simulink model "Correct_ESC_Model_with_Motor_Quadcopter_E2A"  (R2018b)
settings: Solver=VariableStepAuto  StartTime=0.0  StopTime=10  RelTol=1e-3
settings Model: Creator=hermansoyfer  LastModifiedBy=tdarrah
settings SFSimCC: SimUseLocalCustomCode=off
settings RTWCC: RTWUseLocalCustomCode=off
settings CodeAppCC: StateflowObjectComments=on

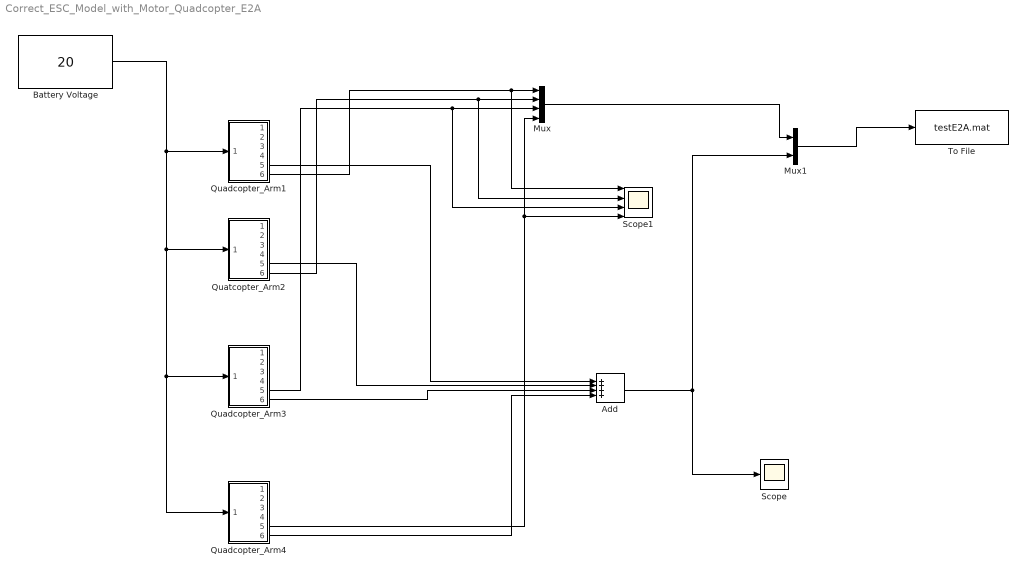
== system Correct_ESC_Model_with_Motor_Quadcopter_E2A ==
  Add : Sum  Inputs=++++
  Battery Voltage : Constant  Value=20
  Mux : Mux
  Mux1 : Mux  Inputs=2
  Quadcopter_Arm1 : Subsystem
  Quadcopter_Arm3 : Subsystem
  Quadcopter_Arm4 : Subsystem
  Quatcopter_Arm2 : Subsystem
  Scope : Scope
  Scope1 : Scope  NumInputPorts=4
  To File : ToFile  Filename=testE2A.mat  MatrixName=Data
  wires:
  Battery Voltage/1 -> Quadcopter_Arm1/1(In1), Quatcopter_Arm2/1(In1), Quadcopter_Arm3/1(In1), Quadcopter_Arm4/1(In1)
  Quadcopter_Arm1/5(M1Current) -> Add/1
  Quatcopter_Arm2/5(M2Current) -> Add/2
  Quadcopter_Arm3/6(M3Current) -> Add/3
  Quadcopter_Arm4/6(M4Current) -> Add/4
  Add/1 -> Mux1/2, Scope/1
  Quadcopter_Arm1/6(M1Voltage) -> Scope1/1, Mux/1
  Quatcopter_Arm2/6(M2Voltatge) -> Scope1/2, Mux/2
  Quadcopter_Arm3/5(M3Voltage) -> Scope1/3, Mux/3
  Quadcopter_Arm4/5(M4Voltage) -> Scope1/4, Mux/4
  Mux/1 -> Mux1/1
  Mux1/1 -> To File/1

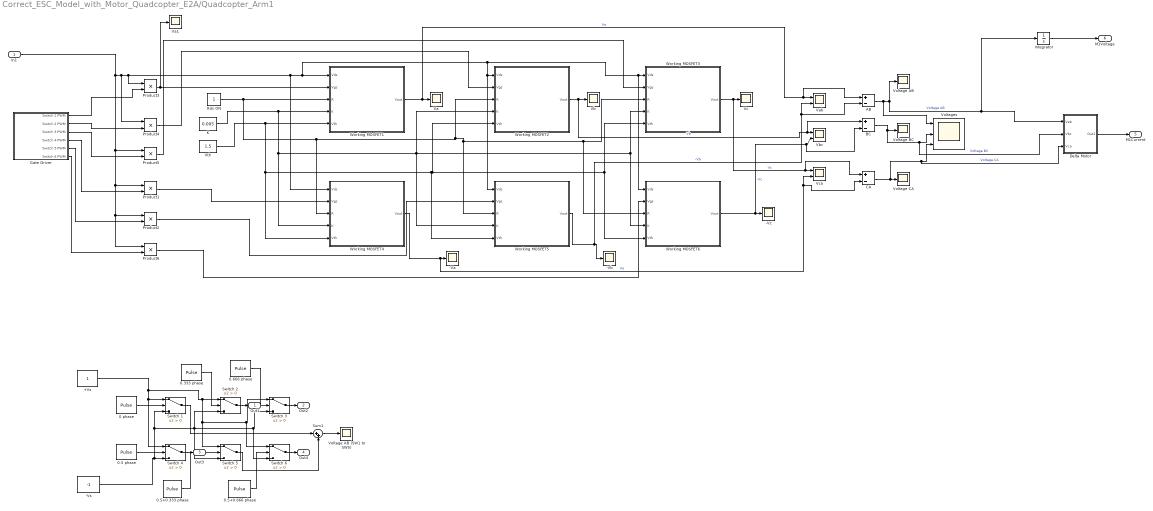
== system Correct_ESC_Model_with_Motor_Quadcopter_E2A/Quadcopter_Arm1 ==
  In1 : Inport
  +Vs : Constant
  -Va : Scope
  -Vb : Scope
  -Vc : Scope
  -Vs : Constant  Value=-1
  0 phase : DiscretePulseGenerator  PulseType=Time based  Period=1  PulseWidth=50
  0.333 phase : DiscretePulseGenerator  PulseType=Time based  Period=1  PulseWidth=50  PhaseDelay=1/3
  0.5 phase : DiscretePulseGenerator  PulseType=Time based  Period=1  PulseWidth=50  PhaseDelay=.5
  0.5+0.333 phase : DiscretePulseGenerator  PulseType=Time based  Period=1  PulseWidth=50  PhaseDelay=0.5 + 1/3
  0.5+0.666 phase : DiscretePulseGenerator  PulseType=Time based  Period=1  PulseWidth=50  PhaseDelay=2/3+0.5
  0.666 phase : DiscretePulseGenerator  PulseType=Time based  Period=1  PulseWidth=50  PhaseDelay=2/3
  AB : Sum  Inputs=+-
  BC : Sum  Inputs=+-
  CA : Sum  Inputs=+-
  Delta Motor : Subsystem
  Gate Driver : Subsystem
  Integrator : Integrator
  K : Constant  Value=0.005
  Product{1..6} (6 alike) : Product
  Rds ON : Constant
  Sum1 : Sum  Inputs=|++
  Switch {1..6} (6 alike) : Switch  Criteria=u2 > Threshold
  Va : Scope
  Va1 : Scope
  Vab : Scope  NumInputPorts=2
  Vb : Scope
  Vbc : Scope  NumInputPorts=2
  Vc : Scope
  Vca : Scope  NumInputPorts=2
  Voltage AB : Scope
  Voltage AB (SW1 to SW5) : Scope
  Voltage BC : Scope
  Voltage CA : Scope
  Voltages : Scope  NumInputPorts=3
  Vth : Constant  Value=1.5
  Working MOSFET1 : MATLAB Function  TreatAsAtomicUnit=on
  Working MOSFET2 : MATLAB Function  TreatAsAtomicUnit=on
  Working MOSFET3 : MATLAB Function  TreatAsAtomicUnit=on
  Working MOSFET4 : MATLAB Function  TreatAsAtomicUnit=on
  Working MOSFET5 : MATLAB Function  TreatAsAtomicUnit=on
  Working MOSFET6 : MATLAB Function  TreatAsAtomicUnit=on
  Out1 : Outport
  Out2 : Outport  Port=2
  Out3 : Outport  Port=3
  Out4 : Outport  Port=4
  M1Current : Outport  Port=5
  M1Voltage : Outport  Port=6
  wires:
  Switch 5/1 -> Sum1/2
  Working MOSFET4/1(Vout) -> CA/2, Vca/2, -Va/1  "Va"
  Working MOSFET6/1(Vout) -> BC/2, Vbc/2, -Vc/1  "-Vc"
  AB/1 -> Voltages/1, Integrator/1, Delta Motor/1(Vab), Voltage AB/1  "Voltage AB"
  In1/1 -> Product6/1, Product2/1, Product1/1, Product5/1, Product4/1, Working MOSFET4/1(Vds), Working MOSFET6/1(Vds), Working MOSFET3/1(Vds), Working MOSFET5/1(Vds), Working MOSFET2/1(Vds), Working MOSFET1/1(Vds), Product3/1
  K/1 -> Working MOSFET4/4(K), Working MOSFET5/4(K), Working MOSFET2/4(K), Working MOSFET6/4(K), Working MOSFET3/4(K), Working MOSFET1/4(K)
  Product5/1 -> Working MOSFET3/2(Vgs)
  0.5+0.333 phase/1 -> Switch 5/2
  Gate Driver/3(Switch 3 PWM) -> Product5/2
  Gate Driver/6(Switch 6 PWM) -> Product6/2
  Working MOSFET5/1(Vout) -> AB/2, Vab/2, -Vb/1  "-Vb"
  Gate Driver/5(Switch 5 PWM) -> Product2/2
  Working MOSFET1/1(Vout) -> AB/1, Vab/1, Va/1  "Va"
  0 phase/1 -> Switch 1/2
  Gate Driver/2(Switch 2 PWM) -> Product4/2
  Gate Driver/4(Switch 4 PWM) -> Product1/2
  BC/1 -> Delta Motor/2(Vbc), Voltages/2, Voltage BC/1  "Voltage BC"
  CA/1 -> Delta Motor/3(Vca), Voltages/3, Voltage CA/1  "Voltage CA"
  Working MOSFET3/1(Vout) -> CA/1, Vca/1, Vc/1  "Vc"
  Vth/1 -> Working MOSFET4/5(Vth), Working MOSFET5/5(Vth), Working MOSFET2/5(Vth), Working MOSFET6/5(Vth), Working MOSFET3/5(Vth), Working MOSFET1/5(Vth)
  Product1/1 -> Working MOSFET4/2(Vgs)
  0.333 phase/1 -> Switch 2/2
  Sum1/1 -> Voltage AB (SW1 to SW5)/1
  0.5 phase/1 -> Switch 4/2
  Switch 1/1 -> Sum1/1
  Working MOSFET2/1(Vout) -> BC/1, Vbc/1, Vb/1  "Vb"
  Switch 6/1 -> Out4/1
  Switch 2/1 -> Out1/1
  Switch 4/1 -> Out3/1
  Product2/1 -> Working MOSFET5/2(Vgs)
  Switch 3/1 -> Out2/1
  +Vs/1 -> Switch 6/1, Switch 3/1, Switch 5/1, Switch 2/1, Switch 4/1, Switch 1/1
  0.666 phase/1 -> Switch 3/2
  0.5+0.666 phase/1 -> Switch 6/2
  -Vs/1 -> Switch 1/3, Switch 6/3, Switch 3/3, Switch 2/3, Switch 5/3, Switch 4/3
  Rds ON/1 -> Working MOSFET1/3(R), Working MOSFET4/3(R), Working MOSFET3/3(R), Working MOSFET6/3(R), Working MOSFET5/3(R), Working MOSFET2/3(R)
  Product4/1 -> Working MOSFET2/2(Vgs)
  Product3/1 -> Working MOSFET1/2(Vgs), Va1/1
  Product6/1 -> Working MOSFET6/2(Vgs)
  Delta Motor/1(Out1) -> M1Current/1
  Integrator/1 -> M1Voltage/1
  Gate Driver/1(Switch 1 PWM) -> Product3/2

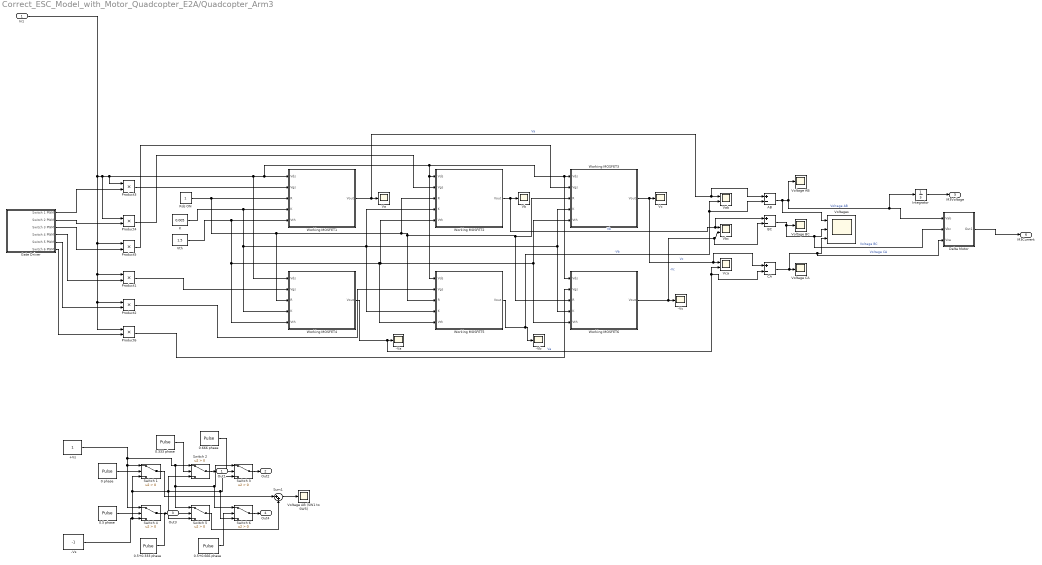
== system Correct_ESC_Model_with_Motor_Quadcopter_E2A/Quadcopter_Arm3 ==
  In1 : Inport
  +Vs : Constant
  -Va : Scope
  -Vb : Scope
  -Vc : Scope
  -Vs : Constant  Value=-1
  0 phase : DiscretePulseGenerator  PulseType=Time based  Period=1  PulseWidth=50
  0.333 phase : DiscretePulseGenerator  PulseType=Time based  Period=1  PulseWidth=50  PhaseDelay=1/3
  0.5 phase : DiscretePulseGenerator  PulseType=Time based  Period=1  PulseWidth=50  PhaseDelay=.5
  0.5+0.333 phase : DiscretePulseGenerator  PulseType=Time based  Period=1  PulseWidth=50  PhaseDelay=0.5 + 1/3
  0.5+0.666 phase : DiscretePulseGenerator  PulseType=Time based  Period=1  PulseWidth=50  PhaseDelay=2/3+0.5
  0.666 phase : DiscretePulseGenerator  PulseType=Time based  Period=1  PulseWidth=50  PhaseDelay=2/3
  AB : Sum  Inputs=+-
  BC : Sum  Inputs=+-
  CA : Sum  Inputs=+-
  Delta Motor : Subsystem
  Gate Driver : Subsystem
  Integrator : Integrator
  K : Constant  Value=0.005
  Product{1..6} (6 alike) : Product
  Rds ON : Constant
  Sum1 : Sum  Inputs=|++
  Switch {1..6} (6 alike) : Switch  Criteria=u2 > Threshold
  Va : Scope
  Vab : Scope  NumInputPorts=2
  Vb : Scope
  Vbc : Scope  NumInputPorts=2
  Vc : Scope
  Vca : Scope  NumInputPorts=2
  Voltage AB : Scope
  Voltage AB (SW1 to SW5) : Scope
  Voltage BC : Scope
  Voltage CA : Scope
  Voltages : Scope  NumInputPorts=3
  Vth : Constant  Value=1.5
  Working MOSFET1 : MATLAB Function  TreatAsAtomicUnit=on
  Working MOSFET2 : MATLAB Function  TreatAsAtomicUnit=on
  Working MOSFET3 : MATLAB Function  TreatAsAtomicUnit=on
  Working MOSFET4 : MATLAB Function  TreatAsAtomicUnit=on
  Working MOSFET5 : MATLAB Function  TreatAsAtomicUnit=on
  Working MOSFET6 : MATLAB Function  TreatAsAtomicUnit=on
  Out1 : Outport
  Out2 : Outport  Port=2
  Out3 : Outport  Port=3
  Out4 : Outport  Port=4
  M3Voltage : Outport  Port=5
  M3Current : Outport  Port=6
  wires:
  Switch 5/1 -> Sum1/2
  Working MOSFET4/1(Vout) -> CA/2, Vca/2, -Va/1  "Va"
  Working MOSFET6/1(Vout) -> BC/2, Vbc/2, -Vc/1  "-Vc"
  AB/1 -> Voltages/1, Integrator/1, Delta Motor/1(Vab), Voltage AB/1  "Voltage AB"
  In1/1 -> Product6/1, Product2/1, Product1/1, Product5/1, Product4/1, Working MOSFET4/1(Vds), Working MOSFET6/1(Vds), Working MOSFET3/1(Vds), Working MOSFET5/1(Vds), Working MOSFET2/1(Vds), Working MOSFET1/1(Vds), Product3/1
  K/1 -> Working MOSFET4/4(K), Working MOSFET5/4(K), Working MOSFET2/4(K), Working MOSFET6/4(K), Working MOSFET3/4(K), Working MOSFET1/4(K)
  Product5/1 -> Working MOSFET3/2(Vgs)
  0.5+0.333 phase/1 -> Switch 5/2
  Gate Driver/3(Switch 3 PWM) -> Product5/2
  Gate Driver/6(Switch 6 PWM) -> Product6/2
  Working MOSFET5/1(Vout) -> AB/2, Vab/2, -Vb/1  "-Vb"
  Gate Driver/5(Switch 5 PWM) -> Product2/2
  Working MOSFET1/1(Vout) -> AB/1, Vab/1, Va/1  "Va"
  0 phase/1 -> Switch 1/2
  Gate Driver/2(Switch 2 PWM) -> Product4/2
  Gate Driver/4(Switch 4 PWM) -> Product1/2
  BC/1 -> Delta Motor/2(Vbc), Voltages/2, Voltage BC/1  "Voltage BC"
  CA/1 -> Delta Motor/3(Vca), Voltages/3, Voltage CA/1  "Voltage CA"
  Working MOSFET3/1(Vout) -> CA/1, Vca/1, Vc/1  "Vc"
  Gate Driver/1(Switch 1 PWM) -> Product3/2
  Vth/1 -> Working MOSFET4/5(Vth), Working MOSFET5/5(Vth), Working MOSFET2/5(Vth), Working MOSFET6/5(Vth), Working MOSFET3/5(Vth), Working MOSFET1/5(Vth)
  Product1/1 -> Working MOSFET4/2(Vgs)
  0.333 phase/1 -> Switch 2/2
  Sum1/1 -> Voltage AB (SW1 to SW5)/1
  0.5 phase/1 -> Switch 4/2
  Switch 1/1 -> Sum1/1
  Working MOSFET2/1(Vout) -> BC/1, Vbc/1, Vb/1  "Vb"
  Switch 6/1 -> Out4/1
  Switch 2/1 -> Out1/1
  Switch 4/1 -> Out3/1
  Product2/1 -> Working MOSFET5/2(Vgs)
  Switch 3/1 -> Out2/1
  +Vs/1 -> Switch 6/1, Switch 3/1, Switch 5/1, Switch 2/1, Switch 4/1, Switch 1/1
  0.666 phase/1 -> Switch 3/2
  0.5+0.666 phase/1 -> Switch 6/2
  -Vs/1 -> Switch 1/3, Switch 6/3, Switch 3/3, Switch 2/3, Switch 5/3, Switch 4/3
  Rds ON/1 -> Working MOSFET1/3(R), Working MOSFET4/3(R), Working MOSFET3/3(R), Working MOSFET6/3(R), Working MOSFET5/3(R), Working MOSFET2/3(R)
  Product4/1 -> Working MOSFET2/2(Vgs)
  Product3/1 -> Working MOSFET1/2(Vgs)
  Product6/1 -> Working MOSFET6/2(Vgs)
  Integrator/1 -> M3Voltage/1
  Delta Motor/1(Out1) -> M3Current/1

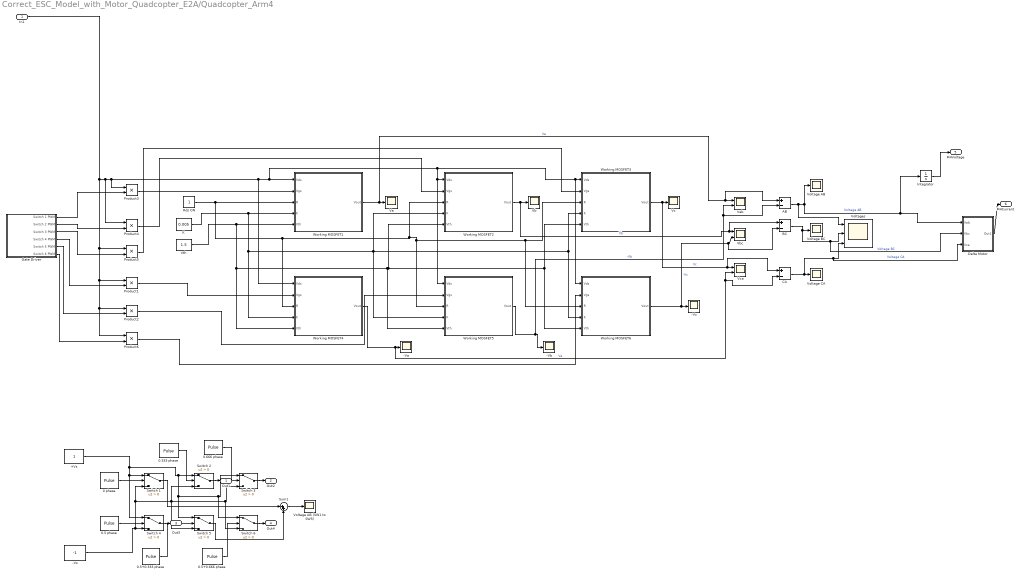
== system Correct_ESC_Model_with_Motor_Quadcopter_E2A/Quadcopter_Arm4 ==
  In1 : Inport
  +Vs : Constant
  -Va : Scope
  -Vb : Scope
  -Vc : Scope
  -Vs : Constant  Value=-1
  0 phase : DiscretePulseGenerator  PulseType=Time based  Period=1  PulseWidth=50
  0.333 phase : DiscretePulseGenerator  PulseType=Time based  Period=1  PulseWidth=50  PhaseDelay=1/3
  0.5 phase : DiscretePulseGenerator  PulseType=Time based  Period=1  PulseWidth=50  PhaseDelay=.5
  0.5+0.333 phase : DiscretePulseGenerator  PulseType=Time based  Period=1  PulseWidth=50  PhaseDelay=0.5 + 1/3
  0.5+0.666 phase : DiscretePulseGenerator  PulseType=Time based  Period=1  PulseWidth=50  PhaseDelay=2/3+0.5
  0.666 phase : DiscretePulseGenerator  PulseType=Time based  Period=1  PulseWidth=50  PhaseDelay=2/3
  AB : Sum  Inputs=+-
  BC : Sum  Inputs=+-
  CA : Sum  Inputs=+-
  Delta Motor : Subsystem
  Gate Driver : Subsystem
  Integrator : Integrator
  K : Constant  Value=0.005
  Product{1..6} (6 alike) : Product
  Rds ON : Constant
  Sum1 : Sum  Inputs=|++
  Switch {1..6} (6 alike) : Switch  Criteria=u2 > Threshold
  Va : Scope
  Vab : Scope  NumInputPorts=2
  Vb : Scope
  Vbc : Scope  NumInputPorts=2
  Vc : Scope
  Vca : Scope  NumInputPorts=2
  Voltage AB : Scope
  Voltage AB (SW1 to SW5) : Scope
  Voltage BC : Scope
  Voltage CA : Scope
  Voltages : Scope  NumInputPorts=3
  Vth : Constant  Value=1.5
  Working MOSFET1 : MATLAB Function  TreatAsAtomicUnit=on
  Working MOSFET2 : MATLAB Function  TreatAsAtomicUnit=on
  Working MOSFET3 : MATLAB Function  TreatAsAtomicUnit=on
  Working MOSFET4 : MATLAB Function  TreatAsAtomicUnit=on
  Working MOSFET5 : MATLAB Function  TreatAsAtomicUnit=on
  Working MOSFET6 : MATLAB Function  TreatAsAtomicUnit=on
  Out1 : Outport
  Out2 : Outport  Port=2
  Out3 : Outport  Port=3
  Out4 : Outport  Port=4
  M4Voltage : Outport  Port=5
  M4Current : Outport  Port=6
  wires:
  Switch 5/1 -> Sum1/2
  Working MOSFET4/1(Vout) -> CA/2, Vca/2, -Va/1  "Va"
  Working MOSFET6/1(Vout) -> BC/2, Vbc/2, -Vc/1  "-Vc"
  AB/1 -> Voltages/1, Integrator/1, Delta Motor/1(Vab), Voltage AB/1  "Voltage AB"
  In1/1 -> Product6/1, Product2/1, Product1/1, Product5/1, Product4/1, Working MOSFET4/1(Vds), Working MOSFET6/1(Vds), Working MOSFET3/1(Vds), Working MOSFET5/1(Vds), Working MOSFET2/1(Vds), Working MOSFET1/1(Vds), Product3/1
  K/1 -> Working MOSFET4/4(K), Working MOSFET5/4(K), Working MOSFET2/4(K), Working MOSFET6/4(K), Working MOSFET3/4(K), Working MOSFET1/4(K)
  Product5/1 -> Working MOSFET3/2(Vgs)
  0.5+0.333 phase/1 -> Switch 5/2
  Gate Driver/3(Switch 3 PWM) -> Product5/2
  Gate Driver/6(Switch 6 PWM) -> Product6/2
  Working MOSFET5/1(Vout) -> AB/2, Vab/2, -Vb/1  "-Vb"
  Gate Driver/5(Switch 5 PWM) -> Product2/2
  Working MOSFET1/1(Vout) -> AB/1, Vab/1, Va/1  "Va"
  0 phase/1 -> Switch 1/2
  Gate Driver/2(Switch 2 PWM) -> Product4/2
  Gate Driver/4(Switch 4 PWM) -> Product1/2
  BC/1 -> Delta Motor/2(Vbc), Voltages/2, Voltage BC/1  "Voltage BC"
  CA/1 -> Delta Motor/3(Vca), Voltages/3, Voltage CA/1  "Voltage CA"
  Working MOSFET3/1(Vout) -> CA/1, Vca/1, Vc/1  "Vc"
  Gate Driver/1(Switch 1 PWM) -> Product3/2
  Vth/1 -> Working MOSFET4/5(Vth), Working MOSFET5/5(Vth), Working MOSFET2/5(Vth), Working MOSFET6/5(Vth), Working MOSFET3/5(Vth), Working MOSFET1/5(Vth)
  Product1/1 -> Working MOSFET4/2(Vgs)
  0.333 phase/1 -> Switch 2/2
  Sum1/1 -> Voltage AB (SW1 to SW5)/1
  0.5 phase/1 -> Switch 4/2
  Switch 1/1 -> Sum1/1
  Working MOSFET2/1(Vout) -> BC/1, Vbc/1, Vb/1  "Vb"
  Switch 6/1 -> Out4/1
  Switch 2/1 -> Out1/1
  Switch 4/1 -> Out3/1
  Product2/1 -> Working MOSFET5/2(Vgs)
  Switch 3/1 -> Out2/1
  +Vs/1 -> Switch 6/1, Switch 3/1, Switch 5/1, Switch 2/1, Switch 4/1, Switch 1/1
  0.666 phase/1 -> Switch 3/2
  0.5+0.666 phase/1 -> Switch 6/2
  -Vs/1 -> Switch 1/3, Switch 6/3, Switch 3/3, Switch 2/3, Switch 5/3, Switch 4/3
  Rds ON/1 -> Working MOSFET1/3(R), Working MOSFET4/3(R), Working MOSFET3/3(R), Working MOSFET6/3(R), Working MOSFET5/3(R), Working MOSFET2/3(R)
  Product4/1 -> Working MOSFET2/2(Vgs)
  Product3/1 -> Working MOSFET1/2(Vgs)
  Product6/1 -> Working MOSFET6/2(Vgs)
  Integrator/1 -> M4Voltage/1
  Delta Motor/1(Out1) -> M4Current/1

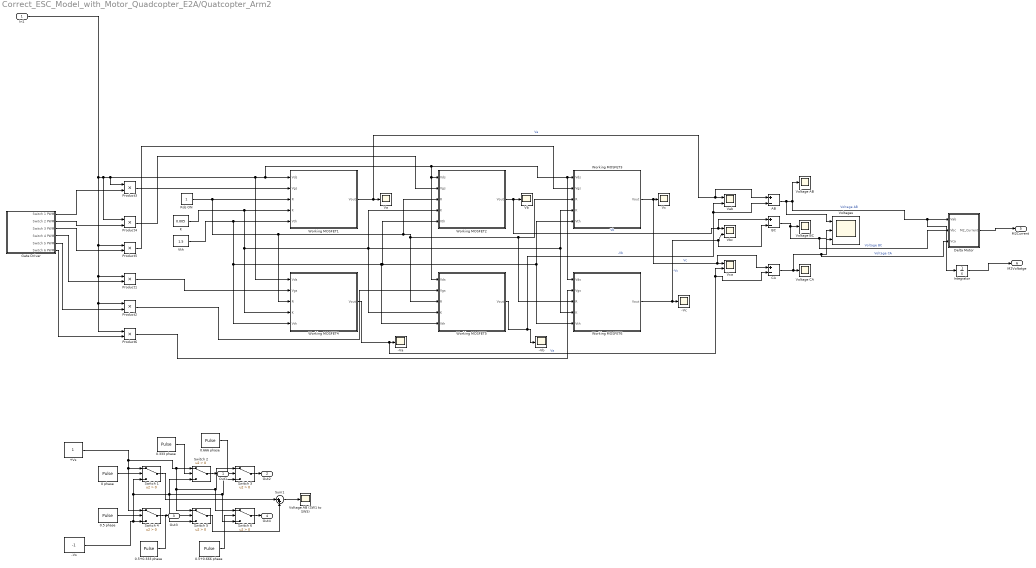
== system Correct_ESC_Model_with_Motor_Quadcopter_E2A/Quatcopter_Arm2 ==
  In1 : Inport
  +Vs : Constant
  -Va : Scope
  -Vb : Scope
  -Vc : Scope
  -Vs : Constant  Value=-1
  0 phase : DiscretePulseGenerator  PulseType=Time based  Period=1  PulseWidth=50
  0.333 phase : DiscretePulseGenerator  PulseType=Time based  Period=1  PulseWidth=50  PhaseDelay=1/3
  0.5 phase : DiscretePulseGenerator  PulseType=Time based  Period=1  PulseWidth=50  PhaseDelay=.5
  0.5+0.333 phase : DiscretePulseGenerator  PulseType=Time based  Period=1  PulseWidth=50  PhaseDelay=0.5 + 1/3
  0.5+0.666 phase : DiscretePulseGenerator  PulseType=Time based  Period=1  PulseWidth=50  PhaseDelay=2/3+0.5
  0.666 phase : DiscretePulseGenerator  PulseType=Time based  Period=1  PulseWidth=50  PhaseDelay=2/3
  AB : Sum  Inputs=+-
  BC : Sum  Inputs=+-
  CA : Sum  Inputs=+-
  Delta Motor : Subsystem
  Gate Driver : Subsystem
  Integrator : Integrator
  K : Constant  Value=0.005
  Product{1..6} (6 alike) : Product
  Rds ON : Constant
  Sum1 : Sum  Inputs=|++
  Switch {1..6} (6 alike) : Switch  Criteria=u2 > Threshold
  Va : Scope
  Vab : Scope  NumInputPorts=2
  Vb : Scope
  Vbc : Scope  NumInputPorts=2
  Vc : Scope
  Vca : Scope  NumInputPorts=2
  Voltage AB : Scope
  Voltage AB (SW1 to SW5) : Scope
  Voltage BC : Scope
  Voltage CA : Scope
  Voltages : Scope  NumInputPorts=3
  Vth : Constant  Value=1.5
  Working MOSFET1 : MATLAB Function  TreatAsAtomicUnit=on
  Working MOSFET2 : MATLAB Function  TreatAsAtomicUnit=on
  Working MOSFET3 : MATLAB Function  TreatAsAtomicUnit=on
  Working MOSFET4 : MATLAB Function  TreatAsAtomicUnit=on
  Working MOSFET5 : MATLAB Function  TreatAsAtomicUnit=on
  Working MOSFET6 : MATLAB Function  TreatAsAtomicUnit=on
  Out1 : Outport
  Out2 : Outport  Port=2
  Out3 : Outport  Port=3
  Out4 : Outport  Port=4
  M2Current : Outport  Port=5
  M2Voltatge : Outport  Port=6
  wires:
  Switch 5/1 -> Sum1/2
  Working MOSFET4/1(Vout) -> CA/2, Vca/2, -Va/1  "Va"
  Working MOSFET6/1(Vout) -> BC/2, Vbc/2, -Vc/1  "-Vc"
  AB/1 -> Voltages/1, Integrator/1, Delta Motor/1(Vab), Voltage AB/1  "Voltage AB"
  In1/1 -> Product6/1, Product2/1, Product1/1, Product5/1, Product4/1, Working MOSFET4/1(Vds), Working MOSFET6/1(Vds), Working MOSFET3/1(Vds), Working MOSFET5/1(Vds), Working MOSFET2/1(Vds), Working MOSFET1/1(Vds), Product3/1
  K/1 -> Working MOSFET4/4(K), Working MOSFET5/4(K), Working MOSFET2/4(K), Working MOSFET6/4(K), Working MOSFET3/4(K), Working MOSFET1/4(K)
  Product5/1 -> Working MOSFET3/2(Vgs)
  0.5+0.333 phase/1 -> Switch 5/2
  Gate Driver/3(Switch 3 PWM) -> Product5/2
  Gate Driver/6(Switch 6 PWM) -> Product6/2
  Working MOSFET5/1(Vout) -> AB/2, Vab/2, -Vb/1  "-Vb"
  Gate Driver/5(Switch 5 PWM) -> Product2/2
  Working MOSFET1/1(Vout) -> AB/1, Vab/1, Va/1  "Va"
  0 phase/1 -> Switch 1/2
  Gate Driver/2(Switch 2 PWM) -> Product4/2
  Gate Driver/4(Switch 4 PWM) -> Product1/2
  BC/1 -> Delta Motor/2(Vbc), Voltages/2, Voltage BC/1  "Voltage BC"
  CA/1 -> Delta Motor/3(Vca), Voltages/3, Voltage CA/1  "Voltage CA"
  Working MOSFET3/1(Vout) -> CA/1, Vca/1, Vc/1  "Vc"
  Gate Driver/1(Switch 1 PWM) -> Product3/2
  Vth/1 -> Working MOSFET4/5(Vth), Working MOSFET5/5(Vth), Working MOSFET2/5(Vth), Working MOSFET6/5(Vth), Working MOSFET3/5(Vth), Working MOSFET1/5(Vth)
  Product1/1 -> Working MOSFET4/2(Vgs)
  0.333 phase/1 -> Switch 2/2
  Sum1/1 -> Voltage AB (SW1 to SW5)/1
  0.5 phase/1 -> Switch 4/2
  Switch 1/1 -> Sum1/1
  Working MOSFET2/1(Vout) -> BC/1, Vbc/1, Vb/1  "Vb"
  Switch 6/1 -> Out4/1
  Switch 2/1 -> Out1/1
  Switch 4/1 -> Out3/1
  Product2/1 -> Working MOSFET5/2(Vgs)
  Switch 3/1 -> Out2/1
  +Vs/1 -> Switch 6/1, Switch 3/1, Switch 5/1, Switch 2/1, Switch 4/1, Switch 1/1
  0.666 phase/1 -> Switch 3/2
  0.5+0.666 phase/1 -> Switch 6/2
  -Vs/1 -> Switch 1/3, Switch 6/3, Switch 3/3, Switch 2/3, Switch 5/3, Switch 4/3
  Rds ON/1 -> Working MOSFET1/3(R), Working MOSFET4/3(R), Working MOSFET3/3(R), Working MOSFET6/3(R), Working MOSFET5/3(R), Working MOSFET2/3(R)
  Product4/1 -> Working MOSFET2/2(Vgs)
  Product3/1 -> Working MOSFET1/2(Vgs)
  Product6/1 -> Working MOSFET6/2(Vgs)
  Delta Motor/1(M2_Current) -> M2Current/1
  Integrator/1 -> M2Voltatge/1

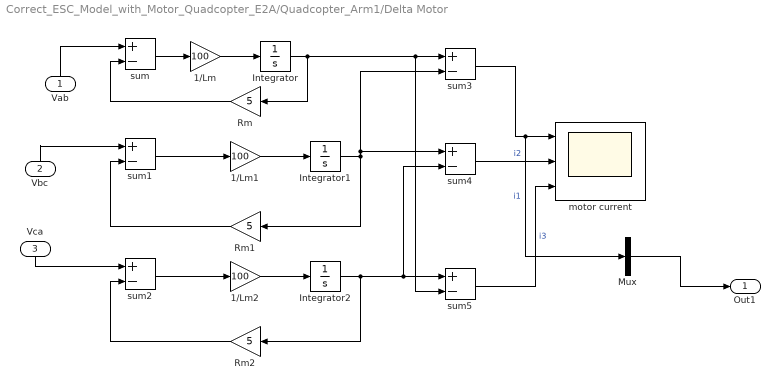
== system Correct_ESC_Model_with_Motor_Quadcopter_E2A/Quadcopter_Arm1/Delta Motor ==
  Vab : Inport
  Vbc : Inport  Port=2
  Vca : Inport  Port=3
  1/Lm : Gain  Gain=100
  1/Lm1 : Gain  Gain=100
  1/Lm2 : Gain  Gain=100
  Integrator : Integrator
  Integrator1 : Integrator
  Integrator2 : Integrator
  Mux : Mux  Inputs=1
  Rm : Gain  Gain=5
  Rm1 : Gain  Gain=5
  Rm2 : Gain  Gain=5
  motor current : Scope  NumInputPorts=3
  sum{,1..5} (6 alike) : Sum  Inputs=+-
  Out1 : Outport
  wires:
  1/Lm2/1 -> Integrator2/1
  Integrator/1 -> sum5/2, sum3/1, Rm/1
  sum3/1 -> Mux/1, motor current/1  "i1"
  Vab/1 -> sum/1
  Rm/1 -> sum/2
  Integrator1/1 -> sum4/1, sum3/2, Rm1/1
  sum1/1 -> 1/Lm1/1
  sum/1 -> 1/Lm/1
  1/Lm1/1 -> Integrator1/1
  Integrator2/1 -> sum5/1, sum4/2, Rm2/1
  1/Lm/1 -> Integrator/1
  sum4/1 -> motor current/2  "i2"
  Rm1/1 -> sum1/2
  Vca/1 -> sum2/1
  sum5/1 -> motor current/3  "i3"
  sum2/1 -> 1/Lm2/1
  Rm2/1 -> sum2/2
  Vbc/1 -> sum1/1
  Mux/1 -> Out1/1

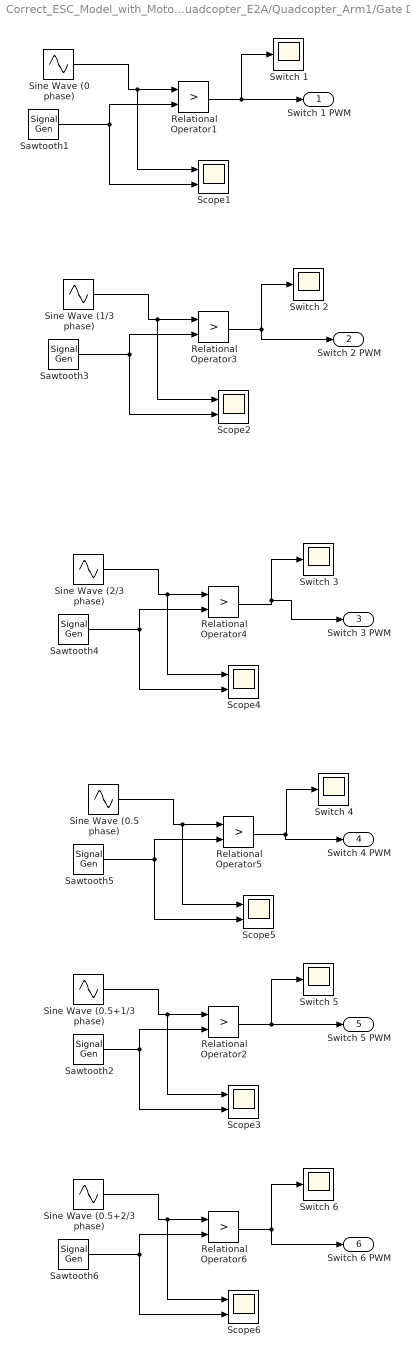
== system Correct_ESC_Model_with_Motor_Quadcopter_E2A/Quadcopter_Arm1/Gate Driver ==
  Relational Operator{1..6} (6 alike) : RelationalOperator  Operator=>  OutDataTypeStr=boolean  RndMeth=Simplest
  Sawtooth{1..6} (6 alike) : SignalGenerator  WaveForm=sawtooth  Frequency=20
  Scope{1..6} (6 alike) : Scope  NumInputPorts=2
  Sine Wave (0 phase) : Sin  Amplitude=0  Frequency=2*pi  SampleTime=0.001
  Sine Wave (0.5 phase) : Sin  Frequency=2*pi  Phase=0.5*(2*pi)  SampleTime=0.001
  Sine Wave (0.5+1/3 phase) : Sin  Frequency=2*pi  Phase=(0.5 + 1/3)*(2*pi)  SampleTime=0.001
  Sine Wave (0.5+2/3 phase) : Sin  Frequency=2*pi  Phase=(2/3 + 0.5)*2*pi  SampleTime=0.001
  Sine Wave (1/3 phase) : Sin  Frequency=2*pi  Phase=(1/3)*(2*pi)  SampleTime=0.001
  Sine Wave (2/3 phase) : Sin  Frequency=2*pi  Phase=(2/3)*(2*pi)  SampleTime=0.001
  Switch {1..6} (6 alike) : Scope
  Switch 1 PWM : Outport
  Switch 2 PWM : Outport  Port=2
  Switch 3 PWM : Outport  Port=3
  Switch 4 PWM : Outport  Port=4
  Switch 5 PWM : Outport  Port=5
  Switch 6 PWM : Outport  Port=6
  wires:
  Relational Operator4/1 -> Switch 3 PWM/1, Switch 3/1
  Sine Wave (1/3 phase)/1 -> Scope2/1, Relational Operator3/1
  Relational Operator6/1 -> Switch 6 PWM/1, Switch 6/1
  Sine Wave (2/3 phase)/1 -> Scope4/1, Relational Operator4/1
  Sawtooth4/1 -> Scope4/2, Relational Operator4/2
  Sawtooth1/1 -> Scope1/2, Relational Operator1/2
  Relational Operator2/1 -> Switch 5 PWM/1, Switch 5/1
  Sine Wave (0.5+2/3 phase)/1 -> Scope6/1, Relational Operator6/1
  Sawtooth5/1 -> Scope5/2, Relational Operator5/2
  Relational Operator1/1 -> Switch 1 PWM/1, Switch 1/1
  Sawtooth6/1 -> Scope6/2, Relational Operator6/2
  Sine Wave (0 phase)/1 -> Scope1/1, Relational Operator1/1
  Sine Wave (0.5 phase)/1 -> Scope5/1, Relational Operator5/1
  Relational Operator3/1 -> Switch 2 PWM/1, Switch 2/1
  Sine Wave (0.5+1/3 phase)/1 -> Scope3/1, Relational Operator2/1
  Sawtooth2/1 -> Scope3/2, Relational Operator2/2
  Sawtooth3/1 -> Scope2/2, Relational Operator3/2
  Relational Operator5/1 -> Switch 4 PWM/1, Switch 4/1

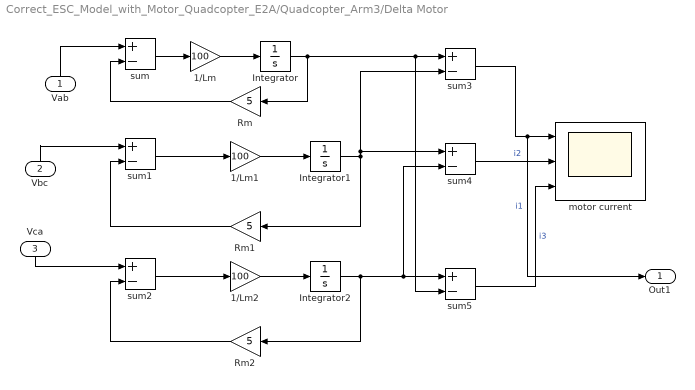
== system Correct_ESC_Model_with_Motor_Quadcopter_E2A/Quadcopter_Arm3/Delta Motor ==
  Vab : Inport
  Vbc : Inport  Port=2
  Vca : Inport  Port=3
  1/Lm : Gain  Gain=100
  1/Lm1 : Gain  Gain=100
  1/Lm2 : Gain  Gain=100
  Integrator : Integrator
  Integrator1 : Integrator
  Integrator2 : Integrator
  Rm : Gain  Gain=5
  Rm1 : Gain  Gain=5
  Rm2 : Gain  Gain=5
  motor current : Scope  NumInputPorts=3
  sum{,1..5} (6 alike) : Sum  Inputs=+-
  Out1 : Outport
  wires:
  1/Lm2/1 -> Integrator2/1
  Integrator/1 -> sum5/2, sum3/1, Rm/1
  sum3/1 -> Out1/1, motor current/1  "i1"
  Vab/1 -> sum/1
  Rm/1 -> sum/2
  Integrator1/1 -> sum4/1, sum3/2, Rm1/1
  sum1/1 -> 1/Lm1/1
  sum/1 -> 1/Lm/1
  1/Lm1/1 -> Integrator1/1
  Integrator2/1 -> sum5/1, sum4/2, Rm2/1
  1/Lm/1 -> Integrator/1
  sum4/1 -> motor current/2  "i2"
  Rm1/1 -> sum1/2
  Vca/1 -> sum2/1
  sum5/1 -> motor current/3  "i3"
  sum2/1 -> 1/Lm2/1
  Rm2/1 -> sum2/2
  Vbc/1 -> sum1/1

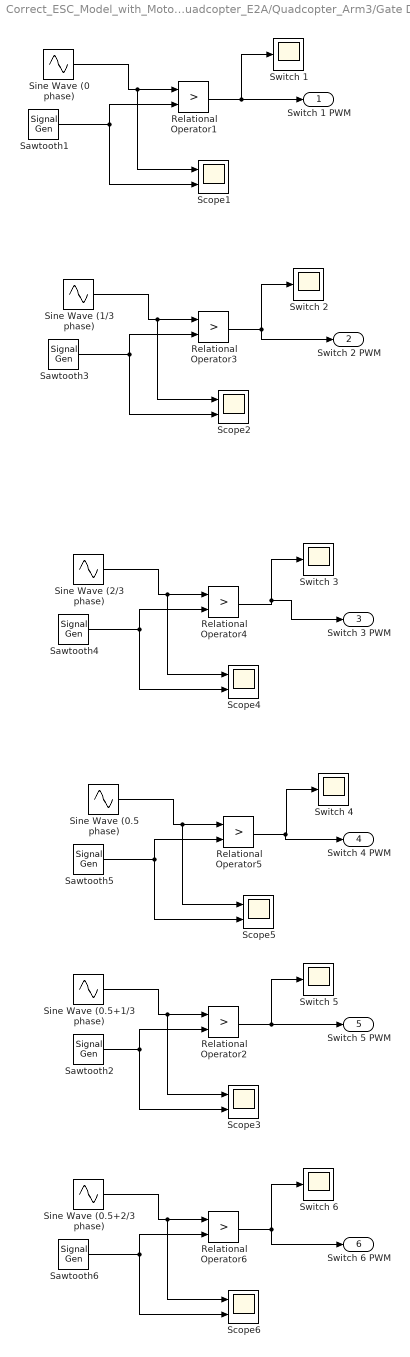
== system Correct_ESC_Model_with_Motor_Quadcopter_E2A/Quadcopter_Arm3/Gate Driver ==
  Relational Operator{1..6} (6 alike) : RelationalOperator  Operator=>  OutDataTypeStr=boolean  RndMeth=Simplest
  Sawtooth{1..6} (6 alike) : SignalGenerator  WaveForm=sawtooth  Frequency=20
  Scope{1..6} (6 alike) : Scope  NumInputPorts=2
  Sine Wave (0 phase) : Sin  Frequency=2*pi  SampleTime=0.001
  Sine Wave (0.5 phase) : Sin  Frequency=2*pi  Phase=0.5*(2*pi)  SampleTime=0.001
  Sine Wave (0.5+1/3 phase) : Sin  Frequency=2*pi  Phase=(0.5 + 1/3)*(2*pi)  SampleTime=0.001
  Sine Wave (0.5+2/3 phase) : Sin  Frequency=2*pi  Phase=(2/3 + 0.5)*2*pi  SampleTime=0.001
  Sine Wave (1/3 phase) : Sin  Frequency=2*pi  Phase=(1/3)*(2*pi)  SampleTime=0.001
  Sine Wave (2/3 phase) : Sin  Frequency=2*pi  Phase=(2/3)*(2*pi)  SampleTime=0.001
  Switch {1..6} (6 alike) : Scope
  Switch 1 PWM : Outport
  Switch 2 PWM : Outport  Port=2
  Switch 3 PWM : Outport  Port=3
  Switch 4 PWM : Outport  Port=4
  Switch 5 PWM : Outport  Port=5
  Switch 6 PWM : Outport  Port=6
  wires:
  Relational Operator4/1 -> Switch 3 PWM/1, Switch 3/1
  Sine Wave (1/3 phase)/1 -> Scope2/1, Relational Operator3/1
  Relational Operator6/1 -> Switch 6 PWM/1, Switch 6/1
  Sine Wave (2/3 phase)/1 -> Scope4/1, Relational Operator4/1
  Sawtooth4/1 -> Scope4/2, Relational Operator4/2
  Sawtooth1/1 -> Scope1/2, Relational Operator1/2
  Relational Operator2/1 -> Switch 5 PWM/1, Switch 5/1
  Sine Wave (0.5+2/3 phase)/1 -> Scope6/1, Relational Operator6/1
  Sawtooth5/1 -> Scope5/2, Relational Operator5/2
  Relational Operator1/1 -> Switch 1 PWM/1, Switch 1/1
  Sawtooth6/1 -> Scope6/2, Relational Operator6/2
  Sine Wave (0 phase)/1 -> Scope1/1, Relational Operator1/1
  Sine Wave (0.5 phase)/1 -> Scope5/1, Relational Operator5/1
  Relational Operator3/1 -> Switch 2 PWM/1, Switch 2/1
  Sine Wave (0.5+1/3 phase)/1 -> Scope3/1, Relational Operator2/1
  Sawtooth2/1 -> Scope3/2, Relational Operator2/2
  Sawtooth3/1 -> Scope2/2, Relational Operator3/2
  Relational Operator5/1 -> Switch 4 PWM/1, Switch 4/1

== system Correct_ESC_Model_with_Motor_Quadcopter_E2A/Quadcopter_Arm4/Delta Motor ==
  Vab : Inport
  Vbc : Inport  Port=2
  Vca : Inport  Port=3
  1/Lm : Gain  Gain=100
  1/Lm1 : Gain  Gain=100
  1/Lm2 : Gain  Gain=100
  Integrator : Integrator
  Integrator1 : Integrator
  Integrator2 : Integrator
  Rm : Gain  Gain=5
  Rm1 : Gain  Gain=5
  Rm2 : Gain  Gain=5
  motor current : Scope  NumInputPorts=3
  sum{,1..5} (6 alike) : Sum  Inputs=+-
  Out1 : Outport
  wires:
  1/Lm2/1 -> Integrator2/1
  Integrator/1 -> sum5/2, sum3/1, Rm/1
  sum3/1 -> Out1/1, motor current/1  "i1"
  Vab/1 -> sum/1
  Rm/1 -> sum/2
  Integrator1/1 -> sum4/1, sum3/2, Rm1/1
  sum1/1 -> 1/Lm1/1
  sum/1 -> 1/Lm/1
  1/Lm1/1 -> Integrator1/1
  Integrator2/1 -> sum5/1, sum4/2, Rm2/1
  1/Lm/1 -> Integrator/1
  sum4/1 -> motor current/2  "i2"
  Rm1/1 -> sum1/2
  Vca/1 -> sum2/1
  sum5/1 -> motor current/3  "i3"
  sum2/1 -> 1/Lm2/1
  Rm2/1 -> sum2/2
  Vbc/1 -> sum1/1

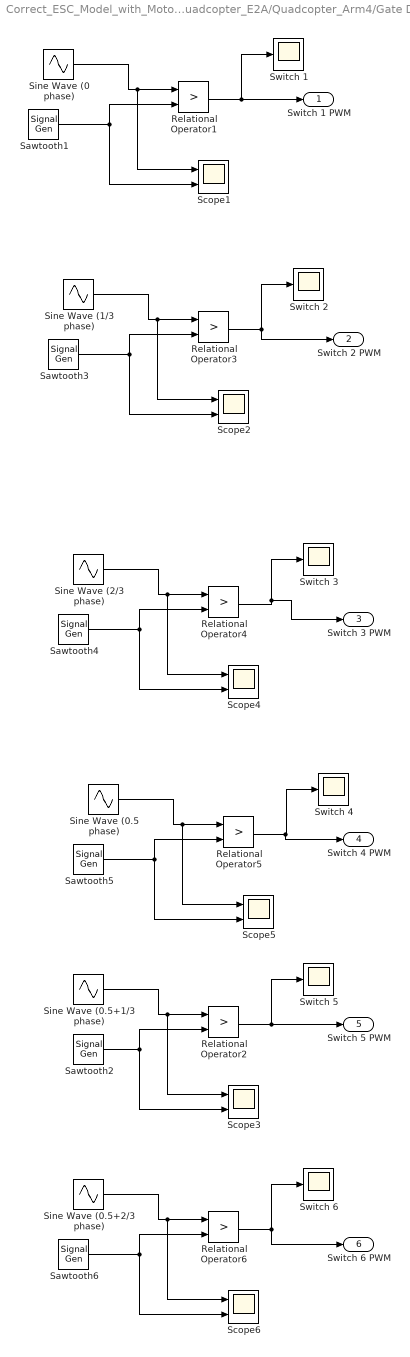
== system Correct_ESC_Model_with_Motor_Quadcopter_E2A/Quadcopter_Arm4/Gate Driver ==
  Relational Operator{1..6} (6 alike) : RelationalOperator  Operator=>  OutDataTypeStr=boolean  RndMeth=Simplest
  Sawtooth{1..6} (6 alike) : SignalGenerator  WaveForm=sawtooth  Frequency=20
  Scope{1..6} (6 alike) : Scope  NumInputPorts=2
  Sine Wave (0 phase) : Sin  Frequency=2*pi  SampleTime=0.001
  Sine Wave (0.5 phase) : Sin  Frequency=2*pi  Phase=0.5*(2*pi)  SampleTime=0.001
  Sine Wave (0.5+1/3 phase) : Sin  Frequency=2*pi  Phase=(0.5 + 1/3)*(2*pi)  SampleTime=0.001
  Sine Wave (0.5+2/3 phase) : Sin  Frequency=2*pi  Phase=(2/3 + 0.5)*2*pi  SampleTime=0.001
  Sine Wave (1/3 phase) : Sin  Frequency=2*pi  Phase=(1/3)*(2*pi)  SampleTime=0.001
  Sine Wave (2/3 phase) : Sin  Frequency=2*pi  Phase=(2/3)*(2*pi)  SampleTime=0.001
  Switch {1..6} (6 alike) : Scope
  Switch 1 PWM : Outport
  Switch 2 PWM : Outport  Port=2
  Switch 3 PWM : Outport  Port=3
  Switch 4 PWM : Outport  Port=4
  Switch 5 PWM : Outport  Port=5
  Switch 6 PWM : Outport  Port=6
  wires:
  Relational Operator4/1 -> Switch 3 PWM/1, Switch 3/1
  Sine Wave (1/3 phase)/1 -> Scope2/1, Relational Operator3/1
  Relational Operator6/1 -> Switch 6 PWM/1, Switch 6/1
  Sine Wave (2/3 phase)/1 -> Scope4/1, Relational Operator4/1
  Sawtooth4/1 -> Scope4/2, Relational Operator4/2
  Sawtooth1/1 -> Scope1/2, Relational Operator1/2
  Relational Operator2/1 -> Switch 5 PWM/1, Switch 5/1
  Sine Wave (0.5+2/3 phase)/1 -> Scope6/1, Relational Operator6/1
  Sawtooth5/1 -> Scope5/2, Relational Operator5/2
  Relational Operator1/1 -> Switch 1 PWM/1, Switch 1/1
  Sawtooth6/1 -> Scope6/2, Relational Operator6/2
  Sine Wave (0 phase)/1 -> Scope1/1, Relational Operator1/1
  Sine Wave (0.5 phase)/1 -> Scope5/1, Relational Operator5/1
  Relational Operator3/1 -> Switch 2 PWM/1, Switch 2/1
  Sine Wave (0.5+1/3 phase)/1 -> Scope3/1, Relational Operator2/1
  Sawtooth2/1 -> Scope3/2, Relational Operator2/2
  Sawtooth3/1 -> Scope2/2, Relational Operator3/2
  Relational Operator5/1 -> Switch 4 PWM/1, Switch 4/1

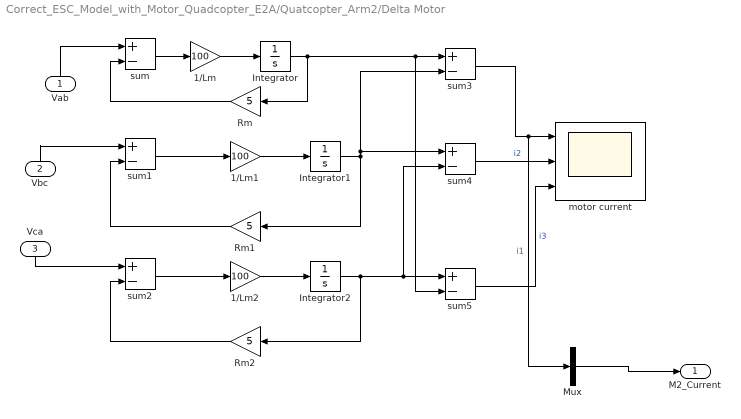
== system Correct_ESC_Model_with_Motor_Quadcopter_E2A/Quatcopter_Arm2/Delta Motor ==
  Vab : Inport
  Vbc : Inport  Port=2
  Vca : Inport  Port=3
  1/Lm : Gain  Gain=100
  1/Lm1 : Gain  Gain=100
  1/Lm2 : Gain  Gain=100
  Integrator : Integrator
  Integrator1 : Integrator
  Integrator2 : Integrator
  Mux : Mux  Inputs=1
  Rm : Gain  Gain=5
  Rm1 : Gain  Gain=5
  Rm2 : Gain  Gain=5
  motor current : Scope  NumInputPorts=3
  sum{,1..5} (6 alike) : Sum  Inputs=+-
  M2_Current : Outport
  wires:
  1/Lm2/1 -> Integrator2/1
  Integrator/1 -> sum5/2, sum3/1, Rm/1
  sum3/1 -> Mux/1, motor current/1  "i1"
  Vab/1 -> sum/1
  Rm/1 -> sum/2
  Integrator1/1 -> sum4/1, sum3/2, Rm1/1
  sum1/1 -> 1/Lm1/1
  sum/1 -> 1/Lm/1
  1/Lm1/1 -> Integrator1/1
  Integrator2/1 -> sum5/1, sum4/2, Rm2/1
  1/Lm/1 -> Integrator/1
  sum4/1 -> motor current/2  "i2"
  Rm1/1 -> sum1/2
  Vca/1 -> sum2/1
  sum5/1 -> motor current/3  "i3"
  sum2/1 -> 1/Lm2/1
  Rm2/1 -> sum2/2
  Vbc/1 -> sum1/1
  Mux/1 -> M2_Current/1

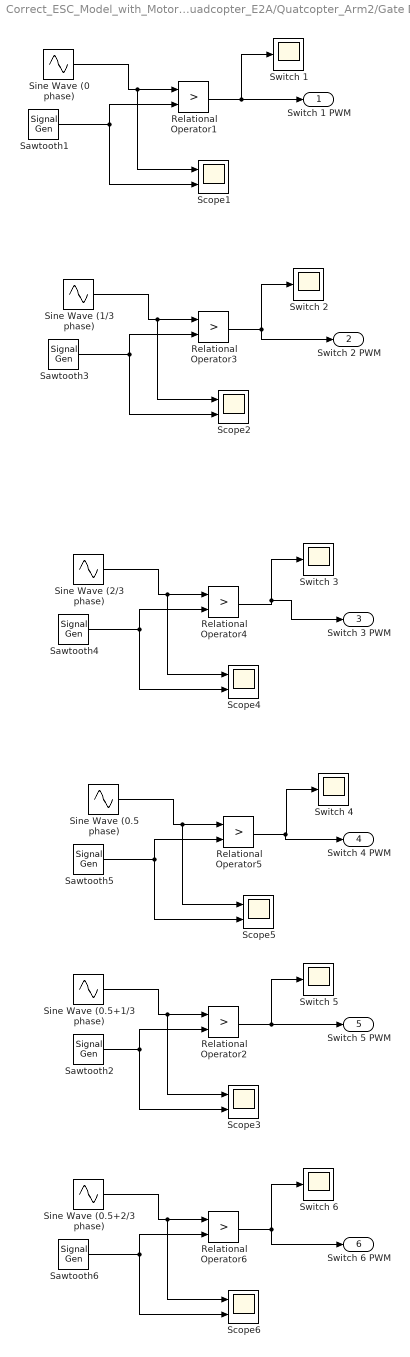
== system Correct_ESC_Model_with_Motor_Quadcopter_E2A/Quatcopter_Arm2/Gate Driver ==
  Relational Operator{1..6} (6 alike) : RelationalOperator  Operator=>  OutDataTypeStr=boolean  RndMeth=Simplest
  Sawtooth{1..6} (6 alike) : SignalGenerator  WaveForm=sawtooth  Frequency=20
  Scope{1..6} (6 alike) : Scope  NumInputPorts=2
  Sine Wave (0 phase) : Sin  Frequency=2*pi  SampleTime=0.001
  Sine Wave (0.5 phase) : Sin  Frequency=2*pi  Phase=0.5*(2*pi)  SampleTime=0.001
  Sine Wave (0.5+1/3 phase) : Sin  Frequency=2*pi  Phase=(0.5 + 1/3)*(2*pi)  SampleTime=0.001
  Sine Wave (0.5+2/3 phase) : Sin  Frequency=2*pi  Phase=(2/3 + 0.5)*2*pi  SampleTime=0.001
  Sine Wave (1/3 phase) : Sin  Frequency=2*pi  Phase=(1/3)*(2*pi)  SampleTime=0.001
  Sine Wave (2/3 phase) : Sin  Frequency=2*pi  Phase=(2/3)*(2*pi)  SampleTime=0.001
  Switch {1..6} (6 alike) : Scope
  Switch 1 PWM : Outport
  Switch 2 PWM : Outport  Port=2
  Switch 3 PWM : Outport  Port=3
  Switch 4 PWM : Outport  Port=4
  Switch 5 PWM : Outport  Port=5
  Switch 6 PWM : Outport  Port=6
  wires:
  Relational Operator4/1 -> Switch 3 PWM/1, Switch 3/1
  Sine Wave (1/3 phase)/1 -> Scope2/1, Relational Operator3/1
  Relational Operator6/1 -> Switch 6 PWM/1, Switch 6/1
  Sine Wave (2/3 phase)/1 -> Scope4/1, Relational Operator4/1
  Sawtooth4/1 -> Scope4/2, Relational Operator4/2
  Sawtooth1/1 -> Scope1/2, Relational Operator1/2
  Relational Operator2/1 -> Switch 5 PWM/1, Switch 5/1
  Sine Wave (0.5+2/3 phase)/1 -> Scope6/1, Relational Operator6/1
  Sawtooth5/1 -> Scope5/2, Relational Operator5/2
  Relational Operator1/1 -> Switch 1 PWM/1, Switch 1/1
  Sawtooth6/1 -> Scope6/2, Relational Operator6/2
  Sine Wave (0 phase)/1 -> Scope1/1, Relational Operator1/1
  Sine Wave (0.5 phase)/1 -> Scope5/1, Relational Operator5/1
  Relational Operator3/1 -> Switch 2 PWM/1, Switch 2/1
  Sine Wave (0.5+1/3 phase)/1 -> Scope3/1, Relational Operator2/1
  Sawtooth2/1 -> Scope3/2, Relational Operator2/2
  Sawtooth3/1 -> Scope2/2, Relational Operator3/2
  Relational Operator5/1 -> Switch 4 PWM/1, Switch 4/1

== matlab function Correct_ESC_Model_with_Motor_Quadcopter_E2A/Quatcopter_Arm2/Working MOSFET1 ==
  data: Vds input; Vgs input; R input; K input; Vth input; Vout output
function Vout   = MOSFET(Vds, Vgs, R, K, Vth)
Ids = 0;
Vd = 0;

    % if gate-source voltage does not exceed threshold, switch is open
    % no current through
    if Vgs <= Vth
        Vd = 0;
        Ids = 0;
        
    % if MOSFET is in linear region    
    elseif Vds<(Vgs-Vth)
        Vd = 20;
        Ids = K*(((Vgs - Vth)*Vds)-((Vds^2)/2));
        
     % if MOSFET is in saturation region   
    elseif (Vgs-Vth)<Vds
         Vd = 20;
         Ids = (K/2)*((Vgs-Vth)^2);         
    end

%calculate voltage output
%this voltage goes to the motor
Vout = Vd - Ids*R;

== matlab function Correct_ESC_Model_with_Motor_Quadcopter_E2A/Quadcopter_Arm1/Working MOSFET2 ==
  data: Vds input; Vgs input; R input; K input; Vth input; Vout output
function Vout   = MOSFET(Vds, Vgs, R, K, Vth)
Ids = 0;
Vd = 0;

    % if gate-source voltage does not exceed threshold, switch is open
    % no current through
    if Vgs <= Vth
        Vd = 0;
        Ids = 0;
        
    % if MOSFET is in linear region    
    elseif Vds<(Vgs-Vth)
        Vd = 20;
        Ids = K*(((Vgs - Vth)*Vds)-((Vds^2)/2));
        
     % if MOSFET is in saturation region   
    elseif (Vgs-Vth)<Vds
         Vd = 20;
         Ids = (K/2)*((Vgs-Vth)^2);         
    end

%calculate voltage output
%this voltage goes to the motor
Vout = Vd - Ids*R;

== matlab function Correct_ESC_Model_with_Motor_Quadcopter_E2A/Quadcopter_Arm1/Working MOSFET3 ==
  data: Vds input; Vgs input; R input; K input; Vth input; Vout output
function Vout   = MOSFET(Vds, Vgs, R, K, Vth)
Ids = 0;
Vd = 0;

    % if gate-source voltage does not exceed threshold, switch is open
    % no current through
    if Vgs <= Vth
        Vd = 0;
        Ids = 0;
        
    % if MOSFET is in linear region    
    elseif Vds<(Vgs-Vth)
        Vd = 20;
        Ids = K*(((Vgs - Vth)*Vds)-((Vds^2)/2));
        
     % if MOSFET is in saturation region   
    elseif (Vgs-Vth)<Vds
         Vd = 20;
         Ids = (K/2)*((Vgs-Vth)^2);         
    end

%calculate voltage output
%this voltage goes to the motor
Vout = Vd - Ids*R;

== matlab function Correct_ESC_Model_with_Motor_Quadcopter_E2A/Quadcopter_Arm1/Working MOSFET4 ==
  data: Vds input; Vgs input; R input; K input; Vth input; Vout output
function Vout   = MOSFET(Vds, Vgs, R, K, Vth)
Ids = 0;
Vd = 0;

    % if gate-source voltage does not exceed threshold, switch is open
    % no current through
    if Vgs <= Vth
        Vd = 0;
        Ids = 0;
        
    % if MOSFET is in linear region    
    elseif Vds<(Vgs-Vth)
        Vd = 20;
        Ids = K*(((Vgs - Vth)*Vds)-((Vds^2)/2));
        
     % if MOSFET is in saturation region   
    elseif (Vgs-Vth)<Vds
         Vd = 20;
         Ids = (K/2)*((Vgs-Vth)^2);         
    end

%calculate voltage output
%this voltage goes to the motor
Vout = Vd - Ids*R;

== matlab function Correct_ESC_Model_with_Motor_Quadcopter_E2A/Quadcopter_Arm1/Working MOSFET5 ==
  data: Vds input; Vgs input; R input; K input; Vth input; Vout output
function Vout   = MOSFET(Vds, Vgs, R, K, Vth)
Ids = 0;
Vd = 0;

    % if gate-source voltage does not exceed threshold, switch is open
    % no current through
    if Vgs <= Vth
        Vd = 0;
        Ids = 0;
        
    % if MOSFET is in linear region    
    elseif Vds<(Vgs-Vth)
        Vd = 20;
        Ids = K*(((Vgs - Vth)*Vds)-((Vds^2)/2));
        
     % if MOSFET is in saturation region   
    elseif (Vgs-Vth)<Vds
         Vd = 20;
         Ids = (K/2)*((Vgs-Vth)^2);         
    end

%calculate voltage output
%this voltage goes to the motor
Vout = Vd - Ids*R;

== matlab function Correct_ESC_Model_with_Motor_Quadcopter_E2A/Quadcopter_Arm1/Working MOSFET6 ==
  data: Vds input; Vgs input; R input; K input; Vth input; Vout output
function Vout   = MOSFET(Vds, Vgs, R, K, Vth)
Ids = 0;
Vd = 0;

    % if gate-source voltage does not exceed threshold, switch is open
    % no current through
    if Vgs <= Vth
        Vd = 0;
        Ids = 0;
        
    % if MOSFET is in linear region    
    elseif Vds<(Vgs-Vth)
        Vd = 20;
        Ids = K*(((Vgs - Vth)*Vds)-((Vds^2)/2));
        
     % if MOSFET is in saturation region   
    elseif (Vgs-Vth)<Vds
         Vd = 20;
         Ids = (K/2)*((Vgs-Vth)^2);         
    end

%calculate voltage output
%this voltage goes to the motor
Vout = Vd - Ids*R;

== matlab function Correct_ESC_Model_with_Motor_Quadcopter_E2A/Quatcopter_Arm2/Working MOSFET2 ==
  data: Vds input; Vgs input; R input; K input; Vth input; Vout output
function Vout   = MOSFET(Vds, Vgs, R, K, Vth)
Ids = 0;
Vd = 0;

    % if gate-source voltage does not exceed threshold, switch is open
    % no current through
    if Vgs <= Vth
        Vd = 0;
        Ids = 0;
        
    % if MOSFET is in linear region    
    elseif Vds<(Vgs-Vth)
        Vd = 20;
        Ids = K*(((Vgs - Vth)*Vds)-((Vds^2)/2));
        
     % if MOSFET is in saturation region   
    elseif (Vgs-Vth)<Vds
         Vd = 20;
         Ids = (K/2)*((Vgs-Vth)^2);         
    end

%calculate voltage output
%this voltage goes to the motor
Vout = Vd - Ids*R;

== matlab function Correct_ESC_Model_with_Motor_Quadcopter_E2A/Quatcopter_Arm2/Working MOSFET3 ==
  data: Vds input; Vgs input; R input; K input; Vth input; Vout output
function Vout   = MOSFET(Vds, Vgs, R, K, Vth)
Ids = 0;
Vd = 0;

    % if gate-source voltage does not exceed threshold, switch is open
    % no current through
    if Vgs <= Vth
        Vd = 0;
        Ids = 0;
        
    % if MOSFET is in linear region    
    elseif Vds<(Vgs-Vth)
        Vd = 20;
        Ids = K*(((Vgs - Vth)*Vds)-((Vds^2)/2));
        
     % if MOSFET is in saturation region   
    elseif (Vgs-Vth)<Vds
         Vd = 20;
         Ids = (K/2)*((Vgs-Vth)^2);         
    end

%calculate voltage output
%this voltage goes to the motor
Vout = Vd - Ids*R;

== matlab function Correct_ESC_Model_with_Motor_Quadcopter_E2A/Quadcopter_Arm1/Working MOSFET1 ==
  data: Vds input; Vgs input; R input; K input; Vth input; Vout output
function Vout   = MOSFET(Vds, Vgs, R, K, Vth)
Ids = 0;
Vd = 0;

    % if gate-source voltage does not exceed threshold, switch is open
    % no current through
    if Vgs <= Vth
        Vd = 0;
        Ids = 0;
        
    % if MOSFET is in linear region    
    elseif Vds<(Vgs-Vth)
        Vd = 20;
        Ids = K*(((Vgs - Vth)*Vds)-((Vds^2)/2));
        
     % if MOSFET is in saturation region   
    elseif (Vgs-Vth)<Vds
         Vd = 20;
         Ids = (K/2)*((Vgs-Vth)^2);         
    end

%calculate voltage output
%this voltage goes to the motor
Vout = Vd - Ids*R;

== matlab function Correct_ESC_Model_with_Motor_Quadcopter_E2A/Quatcopter_Arm2/Working MOSFET4 ==
  data: Vds input; Vgs input; R input; K input; Vth input; Vout output
function Vout   = MOSFET(Vds, Vgs, R, K, Vth)
Ids = 0;
Vd = 0;

    % if gate-source voltage does not exceed threshold, switch is open
    % no current through
    if Vgs <= Vth
        Vd = 0;
        Ids = 0;
        
    % if MOSFET is in linear region    
    elseif Vds<(Vgs-Vth)
        Vd = 20;
        Ids = K*(((Vgs - Vth)*Vds)-((Vds^2)/2));
        
     % if MOSFET is in saturation region   
    elseif (Vgs-Vth)<Vds
         Vd = 20;
         Ids = (K/2)*((Vgs-Vth)^2);         
    end

%calculate voltage output
%this voltage goes to the motor
Vout = Vd - Ids*R;

== matlab function Correct_ESC_Model_with_Motor_Quadcopter_E2A/Quatcopter_Arm2/Working MOSFET5 ==
  data: Vds input; Vgs input; R input; K input; Vth input; Vout output
function Vout   = MOSFET(Vds, Vgs, R, K, Vth)
Ids = 0;
Vd = 0;

    % if gate-source voltage does not exceed threshold, switch is open
    % no current through
    if Vgs <= Vth
        Vd = 0;
        Ids = 0;
        
    % if MOSFET is in linear region    
    elseif Vds<(Vgs-Vth)
        Vd = 20;
        Ids = K*(((Vgs - Vth)*Vds)-((Vds^2)/2));
        
     % if MOSFET is in saturation region   
    elseif (Vgs-Vth)<Vds
         Vd = 20;
         Ids = (K/2)*((Vgs-Vth)^2);         
    end

%calculate voltage output
%this voltage goes to the motor
Vout = Vd - Ids*R;

== matlab function Correct_ESC_Model_with_Motor_Quadcopter_E2A/Quatcopter_Arm2/Working MOSFET6 ==
  data: Vds input; Vgs input; R input; K input; Vth input; Vout output
function Vout   = MOSFET(Vds, Vgs, R, K, Vth)
Ids = 0;
Vd = 0;

    % if gate-source voltage does not exceed threshold, switch is open
    % no current through
    if Vgs <= Vth
        Vd = 0;
        Ids = 0;
        
    % if MOSFET is in linear region    
    elseif Vds<(Vgs-Vth)
        Vd = 20;
        Ids = K*(((Vgs - Vth)*Vds)-((Vds^2)/2));
        
     % if MOSFET is in saturation region   
    elseif (Vgs-Vth)<Vds
         Vd = 20;
         Ids = (K/2)*((Vgs-Vth)^2);         
    end

%calculate voltage output
%this voltage goes to the motor
Vout = Vd - Ids*R;

== matlab function Correct_ESC_Model_with_Motor_Quadcopter_E2A/Quadcopter_Arm3/Working MOSFET1 ==
  data: Vds input; Vgs input; R input; K input; Vth input; Vout output
function Vout   = MOSFET(Vds, Vgs, R, K, Vth)
Ids = 0;
Vd = 0;

    % if gate-source voltage does not exceed threshold, switch is open
    % no current through
    if Vgs <= Vth
        Vd = 0;
        Ids = 0;
        
    % if MOSFET is in linear region    
    elseif Vds<(Vgs-Vth)
        Vd = 20;
        Ids = K*(((Vgs - Vth)*Vds)-((Vds^2)/2));
        
     % if MOSFET is in saturation region   
    elseif (Vgs-Vth)<Vds
         Vd = 20;
         Ids = (K/2)*((Vgs-Vth)^2);         
    end

%calculate voltage output
%this voltage goes to the motor
Vout = Vd - Ids*R;

== matlab function Correct_ESC_Model_with_Motor_Quadcopter_E2A/Quadcopter_Arm3/Working MOSFET2 ==
  data: Vds input; Vgs input; R input; K input; Vth input; Vout output
function Vout   = MOSFET(Vds, Vgs, R, K, Vth)
Ids = 0;
Vd = 0;

    % if gate-source voltage does not exceed threshold, switch is open
    % no current through
    if Vgs <= Vth
        Vd = 0;
        Ids = 0;
        
    % if MOSFET is in linear region    
    elseif Vds<(Vgs-Vth)
        Vd = 20;
        Ids = K*(((Vgs - Vth)*Vds)-((Vds^2)/2));
        
     % if MOSFET is in saturation region   
    elseif (Vgs-Vth)<Vds
         Vd = 20;
         Ids = (K/2)*((Vgs-Vth)^2);         
    end

%calculate voltage output
%this voltage goes to the motor
Vout = Vd - Ids*R;

== matlab function Correct_ESC_Model_with_Motor_Quadcopter_E2A/Quadcopter_Arm3/Working MOSFET3 ==
  data: Vds input; Vgs input; R input; K input; Vth input; Vout output
function Vout   = MOSFET(Vds, Vgs, R, K, Vth)
Ids = 0;
Vd = 0;

    % if gate-source voltage does not exceed threshold, switch is open
    % no current through
    if Vgs <= Vth
        Vd = 0;
        Ids = 0;
        
    % if MOSFET is in linear region    
    elseif Vds<(Vgs-Vth)
        Vd = 20;
        Ids = K*(((Vgs - Vth)*Vds)-((Vds^2)/2));
        
     % if MOSFET is in saturation region   
    elseif (Vgs-Vth)<Vds
         Vd = 20;
         Ids = (K/2)*((Vgs-Vth)^2);         
    end

%calculate voltage output
%this voltage goes to the motor
Vout = Vd - Ids*R;

== matlab function Correct_ESC_Model_with_Motor_Quadcopter_E2A/Quadcopter_Arm3/Working MOSFET4 ==
  data: Vds input; Vgs input; R input; K input; Vth input; Vout output
function Vout   = MOSFET(Vds, Vgs, R, K, Vth)
Ids = 0;
Vd = 0;

    % if gate-source voltage does not exceed threshold, switch is open
    % no current through
    if Vgs <= Vth
        Vd = 0;
        Ids = 0;
        
    % if MOSFET is in linear region    
    elseif Vds<(Vgs-Vth)
        Vd = 20;
        Ids = K*(((Vgs - Vth)*Vds)-((Vds^2)/2));
        
     % if MOSFET is in saturation region   
    elseif (Vgs-Vth)<Vds
         Vd = 20;
         Ids = (K/2)*((Vgs-Vth)^2);         
    end

%calculate voltage output
%this voltage goes to the motor
Vout = Vd - Ids*R;

== matlab function Correct_ESC_Model_with_Motor_Quadcopter_E2A/Quadcopter_Arm3/Working MOSFET5 ==
  data: Vds input; Vgs input; R input; K input; Vth input; Vout output
function Vout   = MOSFET(Vds, Vgs, R, K, Vth)
Ids = 0;
Vd = 0;

    % if gate-source voltage does not exceed threshold, switch is open
    % no current through
    if Vgs <= Vth
        Vd = 0;
        Ids = 0;
        
    % if MOSFET is in linear region    
    elseif Vds<(Vgs-Vth)
        Vd = 20;
        Ids = K*(((Vgs - Vth)*Vds)-((Vds^2)/2));
        
     % if MOSFET is in saturation region   
    elseif (Vgs-Vth)<Vds
         Vd = 20;
         Ids = (K/2)*((Vgs-Vth)^2);         
    end

%calculate voltage output
%this voltage goes to the motor
Vout = Vd - Ids*R;

== matlab function Correct_ESC_Model_with_Motor_Quadcopter_E2A/Quadcopter_Arm3/Working MOSFET6 ==
  data: Vds input; Vgs input; R input; K input; Vth input; Vout output
function Vout   = MOSFET(Vds, Vgs, R, K, Vth)
Ids = 0;
Vd = 0;

    % if gate-source voltage does not exceed threshold, switch is open
    % no current through
    if Vgs <= Vth
        Vd = 0;
        Ids = 0;
        
    % if MOSFET is in linear region    
    elseif Vds<(Vgs-Vth)
        Vd = 20;
        Ids = K*(((Vgs - Vth)*Vds)-((Vds^2)/2));
        
     % if MOSFET is in saturation region   
    elseif (Vgs-Vth)<Vds
         Vd = 20;
         Ids = (K/2)*((Vgs-Vth)^2);         
    end

%calculate voltage output
%this voltage goes to the motor
Vout = Vd - Ids*R;

== matlab function Correct_ESC_Model_with_Motor_Quadcopter_E2A/Quadcopter_Arm4/Working MOSFET1 ==
  data: Vds input; Vgs input; R input; K input; Vth input; Vout output
function Vout   = MOSFET(Vds, Vgs, R, K, Vth)
Ids = 0;
Vd = 0;

    % if gate-source voltage does not exceed threshold, switch is open
    % no current through
    if Vgs <= Vth
        Vd = 0;
        Ids = 0;
        
    % if MOSFET is in linear region    
    elseif Vds<(Vgs-Vth)
        Vd = 20;
        Ids = K*(((Vgs - Vth)*Vds)-((Vds^2)/2));
        
     % if MOSFET is in saturation region   
    elseif (Vgs-Vth)<Vds
         Vd = 20;
         Ids = (K/2)*((Vgs-Vth)^2);         
    end

%calculate voltage output
%this voltage goes to the motor
Vout = Vd - Ids*R;

== matlab function Correct_ESC_Model_with_Motor_Quadcopter_E2A/Quadcopter_Arm4/Working MOSFET2 ==
  data: Vds input; Vgs input; R input; K input; Vth input; Vout output
function Vout   = MOSFET(Vds, Vgs, R, K, Vth)
Ids = 0;
Vd = 0;

    % if gate-source voltage does not exceed threshold, switch is open
    % no current through
    if Vgs <= Vth
        Vd = 0;
        Ids = 0;
        
    % if MOSFET is in linear region    
    elseif Vds<(Vgs-Vth)
        Vd = 20;
        Ids = K*(((Vgs - Vth)*Vds)-((Vds^2)/2));
        
     % if MOSFET is in saturation region   
    elseif (Vgs-Vth)<Vds
         Vd = 20;
         Ids = (K/2)*((Vgs-Vth)^2);         
    end

%calculate voltage output
%this voltage goes to the motor
Vout = Vd - Ids*R;

== matlab function Correct_ESC_Model_with_Motor_Quadcopter_E2A/Quadcopter_Arm4/Working MOSFET3 ==
  data: Vds input; Vgs input; R input; K input; Vth input; Vout output
function Vout   = MOSFET(Vds, Vgs, R, K, Vth)
Ids = 0;
Vd = 0;

    % if gate-source voltage does not exceed threshold, switch is open
    % no current through
    if Vgs <= Vth
        Vd = 0;
        Ids = 0;
        
    % if MOSFET is in linear region    
    elseif Vds<(Vgs-Vth)
        Vd = 20;
        Ids = K*(((Vgs - Vth)*Vds)-((Vds^2)/2));
        
     % if MOSFET is in saturation region   
    elseif (Vgs-Vth)<Vds
         Vd = 20;
         Ids = (K/2)*((Vgs-Vth)^2);         
    end

%calculate voltage output
%this voltage goes to the motor
Vout = Vd - Ids*R;

== matlab function Correct_ESC_Model_with_Motor_Quadcopter_E2A/Quadcopter_Arm4/Working MOSFET4 ==
  data: Vds input; Vgs input; R input; K input; Vth input; Vout output
function Vout   = MOSFET(Vds, Vgs, R, K, Vth)
Ids = 0;
Vd = 0;

    % if gate-source voltage does not exceed threshold, switch is open
    % no current through
    if Vgs <= Vth
        Vd = 0;
        Ids = 0;
        
    % if MOSFET is in linear region    
    elseif Vds<(Vgs-Vth)
        Vd = 20;
        Ids = K*(((Vgs - Vth)*Vds)-((Vds^2)/2));
        
     % if MOSFET is in saturation region   
    elseif (Vgs-Vth)<Vds
         Vd = 20;
         Ids = (K/2)*((Vgs-Vth)^2);         
    end

%calculate voltage output
%this voltage goes to the motor
Vout = Vd - Ids*R;

== matlab function Correct_ESC_Model_with_Motor_Quadcopter_E2A/Quadcopter_Arm4/Working MOSFET5 ==
  data: Vds input; Vgs input; R input; K input; Vth input; Vout output
function Vout   = MOSFET(Vds, Vgs, R, K, Vth)
Ids = 0;
Vd = 0;

    % if gate-source voltage does not exceed threshold, switch is open
    % no current through
    if Vgs <= Vth
        Vd = 0;
        Ids = 0;
        
    % if MOSFET is in linear region    
    elseif Vds<(Vgs-Vth)
        Vd = 20;
        Ids = K*(((Vgs - Vth)*Vds)-((Vds^2)/2));
        
     % if MOSFET is in saturation region   
    elseif (Vgs-Vth)<Vds
         Vd = 20;
         Ids = (K/2)*((Vgs-Vth)^2);         
    end

%calculate voltage output
%this voltage goes to the motor
Vout = Vd - Ids*R;

== matlab function Correct_ESC_Model_with_Motor_Quadcopter_E2A/Quadcopter_Arm4/Working MOSFET6 ==
  data: Vds input; Vgs input; R input; K input; Vth input; Vout output
function Vout   = MOSFET(Vds, Vgs, R, K, Vth)
Ids = 0;
Vd = 0;

    % if gate-source voltage does not exceed threshold, switch is open
    % no current through
    if Vgs <= Vth
        Vd = 0;
        Ids = 0;
        
    % if MOSFET is in linear region    
    elseif Vds<(Vgs-Vth)
        Vd = 20;
        Ids = K*(((Vgs - Vth)*Vds)-((Vds^2)/2));
        
     % if MOSFET is in saturation region   
    elseif (Vgs-Vth)<Vds
         Vd = 20;
         Ids = (K/2)*((Vgs-Vth)^2);         
    end

%calculate voltage output
%this voltage goes to the motor
Vout = Vd - Ids*R;
